simulink library "APST_Lib"  (R2016a)
settings: Solver=ode45  StartTime=0.0  StopTime=10.0  RelTol=1e-3
undefined symbols (not defined in the file or in its folder): ACM, COMP_MAP, rev_comms_sink
libraries: APST_Lib x97
(part 6 of 6)

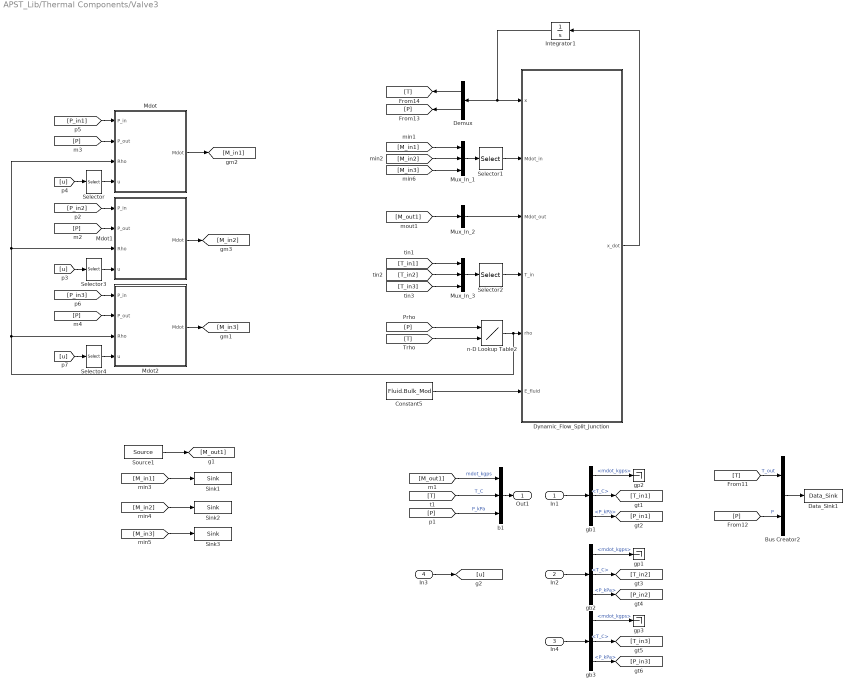
== system APST_Lib/Thermal Components/Valve3 ==
  In1 : Inport
  In2 : Inport  Port=2
  In4 : Inport  Port=3
  In3 : Inport  Port=4
  Bus Creator2 : BusCreator  Inputs=2
  Constant5 : Constant  Value=Fluid.Bulk_Mod
  Data_Sink1 : APST_Lib/Support Components/Data_Sink
  Demux : Demux  Outputs=2
  Dynamic_Flow_Split_Junction : MATLAB Function  TreatAsAtomicUnit=on
  Integrator1 : Integrator  InitialCondition=[T_init P_init]
  Mdot : MATLAB Function  TreatAsAtomicUnit=on
  Mdot1 : MATLAB Function  TreatAsAtomicUnit=on
  Mdot2 : MATLAB Function  TreatAsAtomicUnit=on
  Mux_In_1 : Mux  Inputs=3
  Mux_In_2 : Mux  Inputs=1
  Mux_In_3 : Mux  Inputs=3
  Selector : Selector  InputPortWidth=3  IndexOptions=Index vector (dialog)  Indices=[1]  OutputSizes=1
  Selector1 : Selector  InputPortWidth=3  IndexOptions=Index vector (dialog)  Indices=[1 2 3 ]  OutputSizes=1
  Selector2 : Selector  InputPortWidth=3  IndexOptions=Index vector (dialog)  Indices=[1 2 3 ]  OutputSizes=1
  Selector3 : Selector  InputPortWidth=3  IndexOptions=Index vector (dialog)  Indices=2  OutputSizes=1
  Selector4 : Selector  InputPortWidth=3  IndexOptions=Index vector (dialog)  Indices=3  OutputSizes=1
  Sink1 : APST_Lib/Support Components/Sink
  Sink2 : APST_Lib/Support Components/Sink
  Sink3 : APST_Lib/Support Components/Sink
  Source1 : APST_Lib/Support Components/Source
  b1 : BusCreator  Inputs=3
  gb1 : BusSelector  OutputSignals=mdot_kgps,T_C,P_kPa
  gb2 : BusSelector  OutputSignals=mdot_kgps,T_C,P_kPa
  gb3 : BusSelector  OutputSignals=mdot_kgps,T_C,P_kPa
  gp1 : Terminator
  gp2 : Terminator
  gp3 : Terminator
  n-D Lookup Table2 : Lookup_n-D  BreakpointsForDimension1=Fluid.P  BreakpointsForDimension2=Fluid.T  BreakpointsForDimension3=[5, 7]  Table=Fluid.Rho_pt  ExtrapMethod=Clip  UseLastTableValue=on  RndMeth=Simplest  InputSameDT=on
  Out1 : Outport
  wires:
  [M_in2] -> Sink2/1
  [u] -> Selector3/1
  [u] -> Selector/1
  In3/1 -> [u]
  [M_in2] -> Mux_In_1/2
  [T_in2] -> Mux_In_3/2
  gb2/3 -> [P_in2]  "<P_kPa>"
  In2/1 -> gb2/1
  gb2/1 -> gp1/1  "<mdot_kgps>"
  gb2/2 -> [T_in2]  "<T_C>"
  Mdot1/1(Mdot) -> [M_in2]
  Mdot/1(Mdot) -> [M_in1]
  [P] -> Mdot1/2(P_out)
  [P_in2] -> Mdot1/1(P_in)
  [P] -> Mdot/2(P_out)
  [P_in1] -> Mdot/1(P_in)
  n-D Lookup Table2/1 -> Dynamic_Flow_Split_Junction/5(rho), Mdot2/3(Rho), Mdot/3(Rho), Mdot1/3(Rho)
  Selector2/1 -> Dynamic_Flow_Split_Junction/4(T_in)
  Demux/2 -> [P]
  Demux/1 -> [T]
  [T] -> n-D Lookup Table2/2
  [P] -> n-D Lookup Table2/1
  Constant5/1 -> Dynamic_Flow_Split_Junction/6(E_fluid)
  Selector1/1 -> Dynamic_Flow_Split_Junction/2(Mdot_in)
  Integrator1/1 -> Dynamic_Flow_Split_Junction/1(x), Demux/1
  [P] -> Bus Creator2/2  "P"
  [T] -> Bus Creator2/1  "T_out"
  Bus Creator2/1 -> Data_Sink1/1
  Dynamic_Flow_Split_Junction/1(x_dot) -> Integrator1/1
  [M_in1] -> Sink1/1
  [T_in1] -> Mux_In_3/1
  [M_out1] -> Mux_In_2/1
  [M_in1] -> Mux_In_1/1
  Mux_In_2/1 -> Dynamic_Flow_Split_Junction/3(Mdot_out)
  Mux_In_1/1 -> Selector1/1
  Mux_In_3/1 -> Selector2/1
  gb1/3 -> [P_in1]  "<P_kPa>"
  [P] -> b1/3  "P_kPa"
  In1/1 -> gb1/1
  Source1/1 -> [M_out1]
  gb1/1 -> gp2/1  "<mdot_kgps>"
  [T] -> b1/2  "T_C"
  gb1/2 -> [T_in1]  "<T_C>"
  [M_out1] -> b1/1  "mdot_kgps"
  b1/1 -> Out1/1
  [M_in3] -> Sink3/1
  gb3/3 -> [P_in3]  "<P_kPa>"
  In4/1 -> gb3/1
  gb3/1 -> gp3/1  "<mdot_kgps>"
  gb3/2 -> [T_in3]  "<T_C>"
  Mdot2/1(Mdot) -> [M_in3]
  [u] -> Selector4/1
  [P] -> Mdot2/2(P_out)
  [P_in3] -> Mdot2/1(P_in)
  Selector/1 -> Mdot/4(u)
  Selector3/1 -> Mdot1/4(u)
  Selector4/1 -> Mdot2/4(u)
  [M_in3] -> Mux_In_1/3
  [T_in3] -> Mux_In_3/3

== system APST_Lib/Source & Sinks/Flow Flow Source (Pressure)/Source1 ==
  Out1 : Outport
  wires:
  [NULL] -> Out1/1

== system APST_Lib/Source & Sinks/Flow Source (Mass Flow Rate)/Source1 ==
  Out1 : Outport
  wires:
  [gdata_Thermal_System_BUSM2FSink2] -> Out1/1

== system APST_Lib/Thermal Components/Fluid Tank/Fuel Mass Check ==
  Trigger : TriggerPort  TriggerType=falling  VariantControl=Variant
  Digital Clock : DigitalClock  SampleTime=-1
  MATLAB Function : MATLAB Function  TreatAsAtomicUnit=on
  Terminator : Terminator
  Time of fuel mass going to zero : Display
  wires:
  MATLAB Function/1(y) -> Terminator/1
  Digital Clock/1 -> Time of fuel mass going to zero/1, MATLAB Function/1(u)

== matlab function APST_Lib/Thermal Components/Cold Plate/Cold_Plate ==
  data: x input; Q_load input; x_dot output; P_in input; Mdot_down input; Mdot input; T_in input; H output; mu input; k input; Cp input; Rho input; E_fluid input; f parameter; M_wall parameter; Cp_wall parameter; D parameter; L parameter; t parameter; E parameter; v parameter; KL parameter; dH parameter; H1 parameter
function [x_dot,H]  = Cold_Plate(x,Q_load,P_in,Mdot_down,Mdot,T_in,mu,k,Cp,Rho,E_fluid,f,M_wall,Cp_wall,D,L,t,E,v,KL,dH,H1)

% Constants and Conversions
g       = 9.81;                 % Gravitational acceleration [m/s^2]
A_ht    = pi*L*D;                  % Heat transfer area
V       = L*pi*D^2/4;              % Volume
C_wall  = M_wall*Cp_wall;          % Heat Capacitance (kJ/K)
C_wall  = 1000*C_wall;             % Covnert heat capacitance from kJ/K to J/K
Q_load  = 1000*Q_load;             % Convert load from kW to W
Cp      = 1000*Cp;                 % Convert Cp from J/g*K to J/kg*K
% k       = 1000*k;                  % Convert k from kW/m*K to W/m*K

% Parse states
T       = x(1);                 % Temperature of the tank
P       = x(2);                 % Pressure at bottom of the tank
Tw      = x(3);                 % Wall temperature

% Additional intermediate variable calculations
dP      = (P_in-P)*1000;        % Pressure difference [Pa]
dP      = dP + Rho*g*dH;        % Pressure differential corrected for hieght
% um      = sign(dP)*sqrt_Lip(2*abs(dP)/(Rho*(f*L/D+KL)));    % Fluid velocity [m/s]
% Re      = Rho*um*D/mu;          % Reynolds number
% Pr      = Cp*mu/k;              % Prandtl number (see Incropera, Table 6.2)
% if Re < 2300
%     Nu = 3.66; % (see Incropera, Eq. 8.55)
% else
%     Nu = (f/8)*(Re-1000)*Pr / (1+12.7*(f/8)^.5*(Pr^(2/3)-1)); % (see Incropera, Eq. 8.62)
% end

% Calculate outputs
% H       = PAF*Nu*k/D;               % Heat transfer coefficient (see Incropera, Table 6.2)
H = H1;

% Calculate state derivatives
T_dot   = (Mdot*(T_in-T)+H*A_ht/Cp*(Tw-T))/(V*Rho);     % Outlet temperature 
P_dot   = (Mdot-Mdot_down)/(V*Rho*(1/E_fluid+D*(1-v/2)/(t*E))); % Outlet pressure
Tw_dot  = (Q_load - H*A_ht*(Tw-T))/C_wall;              % Wall temperature

% Mux state derivatives
x_dot  = [T_dot,P_dot,Tw_dot];

end

== matlab function APST_Lib/Thermal Components/Flow Split_Junction/Dynamic_Flow_Split_Junction ==
  data: x input; Mdot_in input; Mdot_out input; T_in input; x_dot output; D parameter; L parameter; t parameter; E parameter; v parameter; rho input; E_fluid input
function x_dot  = Dynamic_Flow_Split_Junction(x,Mdot_in,Mdot_out,T_in,D,L,t,E,v,rho,E_fluid)

% Constants and Conversions
Mdot_in_tot     = sum(Mdot_in);     % Total mass flow rate in
Mdot_out_tot    = sum(Mdot_out);    % Total mass flow rate out
V               = pi*D^2/4*L;       % Volume

% Parse states
T      = x(1);                  % Temperature of the tank
P      = x(2);                  % Pressure at bottom of the tank

% Calculate state derivatives
T_dot = (dot(Mdot_in,T_in)-sum(Mdot_in)*T)/(rho*V);  % Split/Junc temperature
P_dot = (Mdot_in_tot-Mdot_out_tot)/(V*rho*(1/E_fluid+D*(1-v/2)/(t*E))); % Split/Junc pressure

% Mux state derivatives
x_dot  = [T_dot,P_dot];

end

== matlab function APST_Lib/Thermal Components/Heat Exchanger/HX ==
  data: x input; x_dot output; P_in input size=2; Mdot_down input size=2; Mdot input; T_in input size=2; H output; mu input size=2; k input size=2; Cp input size=2; Rho input size=2; E_fluid input size=2; M_wall parameter; Cp_wall parameter; Pass1 parameter; Pass2 parameter; f1 parameter; f2 parameter; KL1 parameter; KL2 parameter; b1 parameter; b2 parameter; W1 parameter; W2 parameter; L1 parameter; L2 parameter; dH1 parameter; dH2 parameter; H1 parameter; H2 parameter
function [x_dot,H]  = HX(x,P_in,Mdot_down,Mdot,T_in,mu,k,Cp,Rho,E_fluid,M_wall,Cp_wall,Pass1,Pass2,f1,f2,KL1,KL2,b1,b2,W1,W2,L1,L2,dH1,dH2,H1, H2)

% Parse data
% P_in1       = P_in(1);
% P_in2       = P_in(2);
Mdot_down1  = Mdot_down(1);
Mdot_down2  = Mdot_down(2);
Mdot1       = Mdot(1);
Mdot2       = Mdot(2);
T_in1       = T_in(1);
T_in2       = T_in(2);
% mu1         = mu(1);
% mu2         = mu(2);
% k1          = k(1);
% k2          = k(2);
Cp1         = Cp(1);
Cp2         = Cp(2);
Rho1        = Rho(1);
Rho2        = Rho(2);
E_fluid1    = E_fluid(1);
E_fluid2    = E_fluid(2);

% Constants and Conversions
Mdot_down1_pass = Mdot_down1/Pass1;
Mdot_down2_pass = Mdot_down2/Pass2;
Mdot1_pass = Mdot1/Pass1;
Mdot2_pass = Mdot2/Pass2;
g        = 9.81;                   % Gravitational acceleration [m/s^2]
A_ht1    = L1*(2*b1+2*W1);         % Heat transfer area
A_ht2    = L2*(2*b2+2*W2);         % Heat transfer area
V1       = L1*b1*W1;               % Volume per pass
V2       = L2*b2*W2;               % Volume per pass
Cp1      = 1000*Cp1;               % Convert Cp from J/g*K to J/kg*K
Cp2      = 1000*Cp2;               % Convert Cp from J/g*K to J/kg*K
% k1       = 1000*k1;                % Convert k from kW/m*K to W/m*K
% k2       = 1000*k2;                % Convert k from kW/m*K to W/m*K
C_wall   = M_wall*Cp_wall;         % Heat Capacitance (kJ/K)
C_wall   = 1000*C_wall;            % Covnert heat capacitance from kJ/K to J/K
% D1       = 4*b1*W1/(2*b1+2*W1);    % Hydraulic diameter (side 1) (see Incropera, Eq. 8.66)
% D2       = 4*b2*W2/(2*b2+2*W2);    % Hydraulic diameter (side 2) (see Incropera, Eq. 8.66)

% Parse states
Tw      = x(1);                 % Wall temperature
% P1      = x(2);                 % Outlet pressure (side 1)
% P2      = x(3);                 % Outlet pressure (side 2)
T1      = x(4);                 % Outlet temperature (side 1)
T2      = x(5);                 % Outlet temperature (side 2)

% Additional intermediate variable calculations
% dP1         = (P_in1-P1)*1000;      % Pressure differential (side 1) [Pa]
% dP2         = (P_in2-P2)*1000;      % Pressure differential (side 2) [Pa]
% dP1         = dP1 + Rho1*g*dH1;     % Pressure differential corrected for hieght
% dP2         = dP2 + Rho2*g*dH2;     % Pressure differential corrected for hieght
% um1         = sign(dP1)*sqrt_Lip(2*abs(dP1)/(Rho1*(f1*L1/D1+KL1)));   % Fluid velocity (side 1) [m/s]
% um2         = sign(dP2)*sqrt_Lip(2*abs(dP2)/(Rho2*(f2*L2/D2+KL2)));   % Fluid velocity (side 2) [m/s]
% Re1         = Rho1*abs(um1)*D1/mu1;      % Reynolds number (side 1)
% Re2         = Rho2*abs(um2)*D2/mu2;      % Reynolds number (side 1)
% Pr1         = Cp1*mu1/k1;           % Prandtl number (side 1) (see Incropera, Table 6.2)
% Pr2         = Cp2*mu2/k2;           % Prandtl number (side 2) (see Incropera, Table 6.2)

% Gneilinski (sp?)
% if Re1 < 2300
%     Nu1 = Nu_lam1; % (inteprolated from Incropera, Table 8.1 in initialization)
% else
%     Nu1 = (f1/8)*(Re1-1000)*Pr1 / (1+12.7*(f1/8)^.5*(Pr1^(2/3)-1)); % (see Incropera, Eq. 8.62)
% end
% if Re2 < 2300
%     Nu2 = Nu_lam2; % (inteprolated from Incropera, Table 8.1 in initialization)
% else
%     Nu2 = (f2/8)*(Re2-1000)*Pr2 / (1+12.7*(f2/8)^.5*(Pr2^(2/3)-1)); % (see Incropera, Eq. 8.62)
% end

% Longo Correlation
% Nu1 = 0.277*Re1^0.766*Pr1^0.333;
% Nu2 = 0.277*Re2^0.766*Pr2^0.333;

% % Manglik Correlation
% Nu1 = 0.44*Re1^0.5*Pr1^0.333;
% Nu2 = 0.44*Re2^0.5*Pr2^0.333;

% Calculate outputs
% H1      = Nu1*k1/D1;        % Heat transfer coefficient (see Incropera, Table 6.2)
% H2      = Nu2*k2/D2;        % Heat transfer coefficient (see Incropera, Table 6.2)
H       = [H1 H2];

% Calculate state derivatives
Tw_dot = ( H1*A_ht1*(T1-Tw) + H2*A_ht2*(T2-Tw) )/C_wall;    % Wall temperature
P1_dot = (Mdot1_pass-Mdot_down1_pass)/(V1*Rho1/E_fluid1);   % Outlet pressure (side 1)
P2_dot = (Mdot2_pass-Mdot_down2_pass)/(V2*Rho2/E_fluid2);   % Outlet pressure (side 2)
Tout1_dot = (Mdot1_pass*(T_in1-T1)+H1*A_ht1/Cp1*(Tw-T1))/(V1*Rho1);   % Outlet temperature (side 1)
Tout2_dot = (Mdot2_pass*(T_in2-T2)+H2*A_ht2/Cp2*(Tw-T2))/(V2*Rho2);   % Outlet temperature (side 2)

% Mux state derivatives
x_dot  = [Tw_dot,P1_dot,P2_dot,Tout1_dot,Tout2_dot];

end

== matlab function APST_Lib/Thermal Components/Fluid Tank/Tank ==
  data: x input; x_dot output; Mdot_in input; Mdot_out input; T_in input; T_amb input; Cp input; Rho input; Q input; H parameter; D parameter; A_sa parameter
function x_dot = Tank(x,Mdot_in,Mdot_out,T_in,T_amb,Cp,Rho,Q,H,D,A_sa)

% Constants and Conversions
A_cross = pi*D^2/4;             % Cross-sectional area
Cp      = 1000*Cp;              % Convert Cp from J/g*K to J/kg*K
g       = 9.81;                 % Gravitational acceleration

% Parse states
T      = x(1);                  % Temperature of the tank
P      = x(2);                  % Pressure at bottom of the tank
M      = x(3);                  % Pressure at bottom of the tank

% Calculate outputs
% h = 1000*(P-Pamb)/(Rho*g);      % Tank height
% M = Rho*A_cross*h;              % Tank mass

% Additional intermediate variable calculations
% A_ht    = pi*h*D;               % Heat transfer area          
A_ht = A_sa;

% Calculate state derivatives
T_dot = (Mdot_in*(T_in-T)-H*A_ht*(T-T_amb)/Cp + Q/Cp)/M; % Tank temperature
% P_dot  = (Mdot_in-Mdot_out)*g/(1000*A_cross);        % Tank pressure
M_dot = (Mdot_in-Mdot_out);

% Mux state derivatives
x_dot  = [T_dot,0,M_dot];

end

== matlab function APST_Lib/Electrical Components/Generator/Generator ==
  data: Omega input; I input; Torque output; V parameter; eta parameter; Q output
function [Torque,Q]   = Generator(Omega,I,V,eta)

% Constants and Conversions

% Parse states

% Additional intermediate variable calculations

% Calculate outputs
Torque = 1/(Omega*eta)*I*V;     % Generator torque (Nm)
Q = (1-eta)*Torque*Omega/1000;       % Generator heat (kW)

% Calculate state derivatives

% Mux state derivatives

end

== matlab function APST_Lib/Thermal Components/Pipe_P_to_P/Pipe_P_to_M ==
  data: x_dot output; x input; T_in input; Mdot input; Rho input; D parameter; L parameter
function x_dot   = Pipe_P_to_M(x,T_in,Mdot,Rho,D,L)

% Constants and Conversions
V      = pi*D^2/4*L;            % Volume

% Parse states
T      = x(1);                  % Temperature of the tank

% Calculate state derivatives
T_dot  = Mdot*(T_in-T)/(V*Rho);  % Pipe outlet temperature

% Mux state derivatives
x_dot  = T_dot;

end

== matlab function APST_Lib/Thermal Components/Pipe_P_to_M/Pipe_P_to_M ==
  data: x_dot output; x input; T_in input; Mdot_down input; Mdot input; Rho input; E_fluid input; D parameter; L parameter; t parameter; E parameter; v parameter
function x_dot  = Pipe_P_to_M(x,T_in,Mdot_down,Mdot,Rho,E_fluid,D,L,t,E,v)

% Constants and Conversions
V       = L*pi*D^2/4;           % Volume

% Parse states
T       = x(1);                 % Temperature at the outlet of pipe
P       = x(2);                 % Pressure at the outlet of pipe

% Calculate state derivatives
T_dot = Mdot*(T_in-T)/(V*Rho);  % Pipe outlet temperature
P_dot = (Mdot-Mdot_down)/(V*Rho*(1/E_fluid+D*(1-v/2)/(t*E)));   % Pipe outlet pressure

% Mux state derivatives
x_dot  = [T_dot,P_dot];

end

== matlab function APST_Lib/Thermal Components/Pipe_P_to_M/Mdot ==
  data: P_in input; P_out input; Mdot output; Rho input; f parameter; D parameter; L parameter; KL parameter; dH parameter
function Mdot = Mdot(P_in,P_out,Rho,f,D,L,KL,dH)

% Constants and Conversions
g           = 9.81;                 % Gravitational acceleration [m/s^2]
A_cross     = pi*D^2/4;             % Cross sectional area
dP          = (P_in-P_out)*1000;    % Pressure differential [Pa]
dP          = dP + Rho*g*dH;        % Pressure differential corrected for hieght
um          = sign(dP)*sqrt_Lip(2*abs(dP)/(Rho*(f*L/D+KL)));    % Fluid velocity [m/s]

% Calculate outputs
Mdot        = um*Rho*A_cross;       % Mass flow rate [kg/s]

end

== matlab function APST_Lib/Air Vehicle Components/Aircraft/Aircraft ==
  data: x input; x_dot output; Thrust_1 input; Thrust_2 input; M_fuel input; M_dry parameter; M_load parameter; rho parameter; A parameter; Cd parameter
function x_dot = Aircraft(x,Thrust_1,Thrust_2,M_fuel,M_dry, M_load, rho, A, Cd)

% Parse states
Vel      = x(1);                  % Velocity of aircraft

% Additional intermediate variable calculations
M_tot  = M_fuel+M_dry+M_load;   % Total mass
Drag   = 0.5*rho*A*Cd*Vel^2;      % Drag force

% Calculate state derivatives
V_dot  = 1/(M_tot)*(Thrust_1+Thrust_2-Drag);    % Velocity

% Mux state derivatives
x_dot  = [V_dot];

end

== matlab function APST_Lib/Thermal Components/Pipe_P_to_P/Mdot ==
  data: P_in input; P_out input; Mdot output; Rho input; f parameter; D parameter; L parameter; KL parameter; dH parameter
function Mdot = Mdot(P_in,P_out,Rho,f,D,L,KL,dH)

% Constants and Conversions
g           = 9.81;                 % Gravitational acceleration [m/s^2]
A_cross     = pi*D^2/4;             % Cross sectional area
dP          = (P_in-P_out)*1000;    % Pressure differential [Pa]
dP          = dP + Rho*g*dH;        % Pressure differential corrected for hieght
um          = sign(dP)*sqrt_Lip(2*abs(dP)/(Rho*(f*L/D+KL)));    % Fluid velocity [m/s]

% Calculate outputs
Mdot        = um*Rho*A_cross;       % Mass flow rate [kg/s]

end

== matlab function APST_Lib/Thermal Components/Cold Plate/Mdot ==
  data: P_in input; P_out input; Mdot output; Rho input; f parameter; D parameter; L parameter; KL parameter; dH parameter
function Mdot = Mdot(P_in,P_out,Rho,f,D,L,KL,dH)

% Constants and Conversions
g           = 9.81;                 % Gravitational acceleration [m/s^2]
A_cross     = pi*D^2/4;             % Cross sectional area
dP          = (P_in-P_out)*1000;    % Pressure differential [Pa]
dP          = dP + Rho*g*dH;        % Pressure differential corrected for hieght
um          = sign(dP)*sqrt_Lip(2*abs(dP)/(Rho*(f*L/D+KL)));    % Fluid velocity [m/s]

% Calculate outputs
Mdot        = um*Rho*A_cross;       % Mass flow rate [kg/s]

end

== matlab function APST_Lib/Thermal Components/Heat Exchanger/Mdot ==
  data: P_in1 input; P_in2 input; Mdot1_tot output; P_out1 input; P_out2 input; Rho1 input; Rho2 input; f1 parameter; f2 parameter; b1 parameter; b2 parameter; W1 parameter; W2 parameter; L1 parameter; L2 parameter; KL1 parameter; KL2 parameter; Mdot2_tot output; Pass1 parameter; Pass2 parameter; dH1 parameter; dH2 parameter
function [Mdot1_tot,Mdot2_tot]   = Mdot(P_in1,P_in2,P_out1,P_out2,Rho1,Rho2,f1,f2,b1,b2,W1,W2,L1,L2,KL1,KL2,Pass1,Pass2,dH1,dH2)

% Constants and Conversions
g           = 9.81;                 % Gravitational acceleration [m/s^2]
D1 = 4*b1*W1/(2*b1+2*W1);           % (see Incropera, Eq. 8.66)
D2 = 4*b2*W2/(2*b2+2*W2);           % (see Incropera, Eq. 8.66)
dP1         = (P_in1-P_out1)*1000;  % Pressure differential (side 1) [Pa]
dP2         = (P_in2-P_out2)*1000;  % Pressure differential (side 2) [Pa]
dP1         = dP1 + Rho1*g*dH1;     % Pressure differential corrected for hieght
dP2         = dP2 + Rho2*g*dH2;     % Pressure differential corrected for hieght
um1         = sign(dP1)*sqrt_Lip(2*abs(dP1)/(Rho1*(f1*L1/D1+KL1))); % Fluid velocity (side 1) [m/s]
um2         = sign(dP2)*sqrt_Lip(2*abs(dP2)/(Rho2*(f2*L2/D2+KL2))); % Fluid velocity (side 2) [m/s]
Mdot1_pass  = um1*Rho1*b1*W1;       % Mass flow rate per pass (side 1) [kg/s]
Mdot2_pass  = um2*Rho2*b2*W2;       % Mass flow rate per pass (side 2) [kg/s]

% Calculate outputs
Mdot1_tot = Mdot1_pass*Pass1;       % Total mass flow rate (side 1) [kg/s]
Mdot2_tot = Mdot2_pass*Pass2;       % Total mass flow rate (side 2) [kg/s]

end

== matlab function APST_Lib/Air Vehicle Components/Engine/Engine ==
  data: x input; Mdot input; Vel input; Torque input; U input; x_dot output; Thrust output; J parameter; Thrust_max parameter; Omega_max parameter; Q_bearings output; alpha parameter; eta parameter
function [x_dot,Thrust,Q_bearings]  = Engine(x,Mdot,Vel,Torque,U,J,Thrust_max,Omega_max, alpha, eta)

% Constants and Conversions

% Parse states
Omega     = x(1);                 % Shaft Speed

% Additional intermediate variable calculations

% Calculate outputs
Thrust    = Thrust_max*(Omega/Omega_max)^3;  % Engine Thrust [N]
Q_burn    = (1-eta)*U*Mdot;           % Heat generation (leaves engine with exhaust) [kW]
Q_bearings = alpha*Omega;               % Bearing heat generation (cooled by oil) [kW]

% Calculate state derivatives
Omega_dot = 1/(J*Omega)*(1000*U*Mdot-Thrust*Vel-Torque*Omega-1000*(Q_burn+Q_bearings));    % Shaft speed 

% Mux state derivatives
x_dot  = [Omega_dot];

end

== matlab function APST_Lib/Thermal Components/Valve3/Dynamic_Flow_Split_Junction ==
  data: x input; Mdot_in input; Mdot_out input; T_in input; x_dot output; D parameter; L parameter; t parameter; E parameter; v parameter; rho input; E_fluid input
function x_dot  = Dynamic_Flow_Split_Junction(x,Mdot_in,Mdot_out,T_in,D,L,t,E,v,rho,E_fluid)

% Constants and Conversions
Mdot_in_tot     = sum(Mdot_in);     % Total mass flow rate in
Mdot_out_tot    = sum(Mdot_out);    % Total mass flow rate out
V               = pi*D^2/4*L;       % Volume

% Parse states
T      = x(1);                  % Temperature of the tank
P      = x(2);                  % Pressure at bottom of the tank

% Calculate state derivatives
T_dot = (dot(Mdot_in,T_in)-sum(Mdot_in)*T)/(rho*V);  % Split/Junc temperature
P_dot = (Mdot_in_tot-Mdot_out_tot)/(V*rho*(1/E_fluid+D*(1-v/2)/(t*E))); % Split/Junc pressure

% Mux state derivatives
x_dot  = [T_dot,P_dot];

end

== matlab function APST_Lib/Thermal Components/Valve3/Mdot ==
  data: P_in input; P_out input; Mdot output; Rho input; u input; D parameter
function Mdot = Mdot(P_in, P_out, Rho, u, D)

% Constants and Conversions
g           = 9.81;                 % Gravitational acceleration [m/s^2]
A_cross     = pi*D^2/4;             % Cross sectional area
dP          = (P_in-P_out)*1000;    % Pressure differential [Pa]
dP          = dP;                   % Pressure differential
um          = sign(dP)*sqrt_Lip(2*abs(dP)/(Rho));    % Fluid velocity [m/s]

% Calculate outputs
Mdot        = u*um*Rho*A_cross;       % Mass flow rate [kg/s]

end

== matlab function APST_Lib/Thermal Components/Flow Split_Junction1/Mdot ==
  data: P_in input; P_out input; Mdot output; Rho input; u input; D parameter
function Mdot = Mdot(P_in, P_out, Rho, u, D)

% Constants and Conversions
g           = 9.81;                 % Gravitational acceleration [m/s^2]
A_cross     = pi*D^2/4;             % Cross sectional area
dP          = (P_in-P_out)*1000;    % Pressure differential [Pa]
dP          = dP;                   % Pressure differential
um          = sign(dP)*sqrt_Lip(2*abs(dP)/(Rho));    % Fluid velocity [m/s]

% Calculate outputs
Mdot        = u*um*Rho*A_cross;       % Mass flow rate [kg/s]

end

== matlab function APST_Lib/Thermal Components/Valve/Mdot ==
  data: P_in input; P_out input; Mdot output; Rho input; f parameter; D parameter; L parameter; KL parameter
function Mdot = Mdot(P_in, P_out, Rho, f, D, L, KL)

% Constants and Conversions
g           = 9.81;                 % Gravitational acceleration [m/s^2]
A_cross     = pi*D^2/4;             % Cross sectional area
dP          = (P_in-P_out)*1000;    % Pressure differential [Pa]
dP          = dP;                   % Pressure differential
um          = sign(dP)*sqrt_Lip(2*abs(dP)/(Rho*(f*L/D+KL)));    % Fluid velocity [m/s]

% Calculate outputs
Mdot        = um*Rho*A_cross;       % Mass flow rate [kg/s]

end

== matlab function APST_Lib/Thermal Components/Valve/Pipe_P_to_M ==
  data: x_dot output; x input; T_in input; Mdot input; Rho input; D parameter; L parameter
function x_dot   = Pipe_P_to_M(x,T_in,Mdot,Rho,D,L)

% Constants and Conversions
V      = pi*D^2/4*L;            % Volume

% Parse states
T      = x(1);                  % Temperature of the tank

% Calculate state derivatives
T_dot  = Mdot*(T_in-T)/(V*Rho);  % Pipe outlet temperature

% Mux state derivatives
x_dot  = T_dot;

end

== matlab function APST_Lib/Thermal Components/Flow Split_Junction1/Mdot1 ==
  data: P_in input; P_out input; Mdot output; Rho input; u input; D parameter
function Mdot = Mdot(P_in, P_out, Rho, u, D)

% Constants and Conversions
g           = 9.81;                 % Gravitational acceleration [m/s^2]
A_cross     = pi*D^2/4;             % Cross sectional area
dP          = (P_in-P_out)*1000;    % Pressure differential [Pa]
dP          = dP;                   % Pressure differential
um          = sign(dP)*sqrt_Lip(2*abs(dP)/(Rho));    % Fluid velocity [m/s]

% Calculate outputs
Mdot        = u*um*Rho*A_cross;       % Mass flow rate [kg/s]

end

== matlab function APST_Lib/Thermal Components/Valve1/Dynamic_Flow_Split_Junction ==
  data: x input; Mdot_in input; Mdot_out input; T_in input; x_dot output; D parameter; L parameter; t parameter; E parameter; v parameter; rho input; E_fluid input
function x_dot  = Dynamic_Flow_Split_Junction(x,Mdot_in,Mdot_out,T_in,D,L,t,E,v,rho,E_fluid)

% Constants and Conversions
Mdot_in_tot     = sum(Mdot_in);     % Total mass flow rate in
Mdot_out_tot    = sum(Mdot_out);    % Total mass flow rate out
V               = pi*D^2/4*L;       % Volume

% Parse states
T      = x(1);                  % Temperature of the tank
P      = x(2);                  % Pressure at bottom of the tank

% Calculate state derivatives
T_dot = (dot(Mdot_in,T_in)-sum(Mdot_in)*T)/(rho*V);  % Split/Junc temperature
P_dot = (Mdot_in_tot-Mdot_out_tot)/(V*rho*(1/E_fluid+D*(1-v/2)/(t*E))); % Split/Junc pressure

% Mux state derivatives
x_dot  = [T_dot,P_dot];

end

== matlab function APST_Lib/Thermal Components/Valve1/Mdot ==
  data: P_in input; P_out input; Mdot output; Rho input; u input; D parameter
function Mdot = Mdot(P_in, P_out, Rho, u, D)

% Constants and Conversions
g           = 9.81;                 % Gravitational acceleration [m/s^2]
A_cross     = pi*D^2/4;             % Cross sectional area
dP          = (P_in-P_out)*1000;    % Pressure differential [Pa]
dP          = dP;                   % Pressure differential
um          = sign(dP)*sqrt_Lip(2*abs(dP)/(Rho));    % Fluid velocity [m/s]

% Calculate outputs
Mdot        = u*um*Rho*A_cross;       % Mass flow rate [kg/s]

end

== matlab function APST_Lib/Thermal Components/Valve1/Mdot1 ==
  data: P_in input; P_out input; Mdot output; Rho input; u input; D parameter
function Mdot = Mdot(P_in, P_out, Rho, u, D)

% Constants and Conversions
g           = 9.81;                 % Gravitational acceleration [m/s^2]
A_cross     = pi*D^2/4;             % Cross sectional area
dP          = (P_in-P_out)*1000;    % Pressure differential [Pa]
dP          = dP;                   % Pressure differential
um          = sign(dP)*sqrt_Lip(2*abs(dP)/(Rho));    % Fluid velocity [m/s]

% Calculate outputs
Mdot        = u*um*Rho*A_cross;       % Mass flow rate [kg/s]

end

== matlab function APST_Lib/Thermal Components/Valve2/Dynamic_Flow_Split_Junction ==
  data: x input; Mdot_in input; Mdot_out input; T_in input; x_dot output; D parameter; L parameter; t parameter; E parameter; v parameter; rho input; E_fluid input
function x_dot  = Dynamic_Flow_Split_Junction(x,Mdot_in,Mdot_out,T_in,D,L,t,E,v,rho,E_fluid)

% Constants and Conversions
Mdot_in_tot     = sum(Mdot_in);     % Total mass flow rate in
Mdot_out_tot    = sum(Mdot_out);    % Total mass flow rate out
V               = pi*D^2/4*L;       % Volume

% Parse states
T      = x(1);                  % Temperature of the tank
P      = x(2);                  % Pressure at bottom of the tank

% Calculate state derivatives
T_dot = (dot(Mdot_in,T_in)-sum(Mdot_in)*T)/(rho*V);  % Split/Junc temperature
P_dot = (Mdot_in_tot-Mdot_out_tot)/(V*rho*(1/E_fluid+D*(1-v/2)/(t*E))); % Split/Junc pressure

% Mux state derivatives
x_dot  = [T_dot,P_dot];

end

== matlab function APST_Lib/Thermal Components/Valve2/Mdot ==
  data: P_in input; P_out input; Mdot output; Rho input; u input; D parameter
function Mdot = Mdot(P_in, P_out, Rho, u, D)

% Constants and Conversions
g           = 9.81;                 % Gravitational acceleration [m/s^2]
A_cross     = pi*D^2/4;             % Cross sectional area
dP          = (P_in-P_out)*1000;    % Pressure differential [Pa]
dP          = dP;                   % Pressure differential
um          = sign(dP)*sqrt_Lip(2*abs(dP)/(Rho));    % Fluid velocity [m/s]

% Calculate outputs
Mdot        = u*um*Rho*A_cross;       % Mass flow rate [kg/s]

end

== matlab function APST_Lib/Thermal Components/Fluid Tank/Fuel Mass Check/MATLAB Function ==
  data: u input; y output
function y = fcn(u)
coder.extrinsic('warning')
coder.extrinsic('gcb')

warning(['Fuel mass has gone to zero. ',...
    'Results may be incorrect after this time.',...
    ' Check in ',gcb])
y = u;

== matlab function APST_Lib/Electrical Components/Battery/Battery ==
  data: x input; V_in input; P input; x_dot output; I_in output; Q output; eta input; C parameter
function [x_dot,I_in,Q]  = Battery(x,V_in,P,eta,C)

% Constants and Conversions

% Parse states
SOC     = x(1);                 % State of charge

% Additional intermediate variable calculations

% Calculate outputs
if P >= 0   % Charge mode
    P_in = 1/eta*P;
    Q = (1-eta)*P_in;
else        % Discharge mode
    P_in = eta*P;
    Q = -(1-eta)*P;
end
I_in = 1000*P_in/V_in;

% Calculate state derivatives
SOC_dot = 1/(1000*C)*P;    % State of charge

% Mux state derivatives
x_dot  = [SOC_dot];

end

== matlab function APST_Lib/Thermal Components/Air Volume/Air_Volume ==
  data: x input; x_dot output; Mdot_in input; Mdot_out input; T_in input; T_amb input; Cp input; Rho input; Q input; H parameter; D parameter; A_sa parameter; V parameter; E_fluid parameter
function x_dot = Air_Volume(x,Mdot_in,Mdot_out,T_in,T_amb,Cp,Rho,Q,H,D,A_sa,V,E_fluid)

% Constants and Conversions
A_cross = pi*D^2/4;             % Cross-sectional area
Cp      = 1000*Cp;              % Convert Cp from J/g*K to J/kg*K
g       = 9.81;                 % Gravitational acceleration

% Parse states
T      = x(1);                  % Temperature of the tank
P      = x(2);                  % Pressure at bottom of the tank
M      = x(3);                  % Pressure at bottom of the tank

% Calculate outputs
% h = 1000*(P-Pamb)/(Rho*g);      % Tank height
% M = Rho*A_cross*h;              % Tank mass

% Additional intermediate variable calculations
% A_ht    = pi*h*D;               % Heat transfer area          
A_ht = A_sa;

% Calculate state derivatives
T_dot = (Mdot_in*(T_in-T)-H*A_ht*(T-T_amb)/Cp + Q/Cp)/M; % Tank temperature
P_dot  = (Mdot_in-Mdot_out)/(V*Rho*(1/E_fluid));        % Tank pressure
% M_dot = (Mdot_in-Mdot_out);

% Mux state derivatives
x_dot  = [T_dot,P_dot,0];

end

== matlab function APST_Lib/Electrical Components/Converter/Converter ==
  data: V_in input; I input; I_in output; V parameter; I0 parameter; Q output; eta_max parameter; eta_min parameter; eta output
function [I_in,Q,eta]   = Converter(V_in,I,V,I0,eta_max, eta_min)

% Constants and Conversions

% Parse states

% Additional intermediate variable calculations
a = -(eta_max-eta_min)/I0^2;
b = 2*(eta_max-eta_min)/I0;
c = eta_min;
eta = a*I^2 + b*I + c;

% Calculate outputs
if V_in > 0
    I_in = 1/(V_in*eta)*I*V;     % Converter torque (Nm)
else
    I_in = 0;
end
Q = (1-eta)*I_in*V_in/1000;       % Converter heat (kW)

% Calculate state derivatives

% Mux state derivatives

end

== matlab function APST_Lib/Thermal Components/Pump1/Pump ==
  data: x input; x_dot output; Mdot output; P_in input; T_in input; V_in input; I output; Mdot_down input; Omega input; E parameter; D parameter; L parameter; Omega_max parameter; DP_max parameter; mdot_max parameter; Q output; alpha parameter; eta output; rho input; cp input
function [x_dot,Mdot,I,Q,eta]= Pump(x,P_in,T_in,V_in,Mdot_down,Omega,E,D,L,Omega_max,DP_max,mdot_max,alpha, rho, cp)

coder.extrinsic('gcb')
% Constants and Conversions
Vol           = L*pi*D^2/4;       % Volume

% Parse states
T       = x(1);                 % Outlet fluid temperature
P       = x(2);                 % Outlet fluid pressure

% Additional intermediate variable calculations
dP      = (P-P_in);             % Pressure difference [kPa]
lambda  = Omega/Omega_max;      % Fraction of max shaft speed [-]
a       = -DP_max/(lambda*mdot_max^2);      % Pump map parameters
c       = lambda*DP_max;                    % Pump map parameters


% Calculate outputs
Q       = alpha*Omega;                       % Heat generation [kW]
if Omega > 0
    Mdot    = max(0,sqrt_Lip((dP-c)/a));                % Mass flow rate [kg/s]
    I       = 1000/V_in*(Mdot*dP/rho+Q);       % Inlet current [A]
    eta     = 1000*(Mdot*dP/rho)/(I*V_in);
else
    Mdot    = 0;                % Mass flow rate [kg/s]
    I       = 0;
    eta     = 0;
end
     
if Omega > Omega_max || (P - P_in) > DP_max || Mdot > mdot_max
%      warning(['Violated maximum values for pump. See ',gcb])
end
% Calculate state derivatives
T_dot   = Mdot*(T_in-T)/(Vol*rho)+Q/(Vol*rho*cp);   % Pump outlet temperature 
P_dot   = (Mdot-Mdot_down)/(Vol*rho/E);     % Pump outlet pressure

% Mux state derivatives
x_dot  = [T_dot,P_dot];

end

== matlab function APST_Lib/Thermal Components/Fan/Pump ==
  data: x input; x_dot output; Mdot output; P_in input; T_in input; V_in input; I output; Mdot_down input; Omega input; E parameter; D parameter; L parameter; Omega_max parameter; DP_max parameter; mdot_max parameter; Q output; alpha parameter; eta output; cp input; rho input
function [x_dot,Mdot,I,Q,eta]= Pump(x,P_in,T_in,V_in,Mdot_down,Omega,E,D,L,Omega_max,DP_max,mdot_max,alpha, cp, rho)


% Constants and Conversions
Vol           = L*pi*D^2/4;       % Volume

% Parse states
T       = x(1);                 % Outlet fluid temperature
P       = x(2);                 % Outlet fluid pressure

% Additional intermediate variable calculations
dP      = (P-P_in);             % Pressure difference [kPa]
lambda  = Omega/Omega_max;      % Fraction of max shaft speed [-]
a       = -DP_max/(lambda*mdot_max^2);      % Pump map parameters
c       = lambda*DP_max;                    % Pump map parameters

% Calculate outputs
Q       = alpha*Omega;                       % Heat generation [kW]
if Omega > 0
    Mdot    = max(0,sqrt_Lip((dP-c)/a));                % Mass flow rate [kg/s]
    I       = 1000/V_in*(Mdot*dP/rho+Q);       % Inlet current [A]
    eta     = 1000*(Mdot*dP/rho)/(I*V_in);
else
    Mdot    = 0;                % Mass flow rate [kg/s]
    I       = 0;
    eta     = 0;
end
         
% Calculate state derivatives
T_dot   = Mdot*(T_in-T)/(Vol*rho)+Q/(Vol*rho*cp);   % Pump outlet temperature 
P_dot   = (Mdot-Mdot_down)/(Vol*rho/E);     % Pump outlet pressure

% Mux state derivatives
x_dot  = [T_dot,P_dot];

end

== matlab function APST_Lib/Thermal Components/Valve3/Mdot1 ==
  data: P_in input; P_out input; Mdot output; Rho input; u input; D parameter
function Mdot = Mdot(P_in, P_out, Rho, u, D)

% Constants and Conversions
g           = 9.81;                 % Gravitational acceleration [m/s^2]
A_cross     = pi*D^2/4;             % Cross sectional area
dP          = (P_in-P_out)*1000;    % Pressure differential [Pa]
dP          = dP;                   % Pressure differential
um          = sign(dP)*sqrt_Lip(2*abs(dP)/(Rho));    % Fluid velocity [m/s]

% Calculate outputs
Mdot        = u*um*Rho*A_cross;       % Mass flow rate [kg/s]

end

== matlab function APST_Lib/Thermal Components/Valve3/Mdot2 ==
  data: P_in input; P_out input; Mdot output; Rho input; u input; D parameter
function Mdot = Mdot(P_in, P_out, Rho, u, D)

% Constants and Conversions
g           = 9.81;                 % Gravitational acceleration [m/s^2]
A_cross     = pi*D^2/4;             % Cross sectional area
dP          = (P_in-P_out)*1000;    % Pressure differential [Pa]
dP          = dP;                   % Pressure differential
um          = sign(dP)*sqrt_Lip(2*abs(dP)/(Rho));    % Fluid velocity [m/s]

% Calculate outputs
Mdot        = u*um*Rho*A_cross;       % Mass flow rate [kg/s]

end
